simulink model "Lab1_adaptive"  (R2022b)
settings: Solver=VariableStepAuto  StartTime=0.0  StopTime=t  MaxStep=0.01  RelTol=1e-3
undefined symbols (not defined in the file): gamma, lambda, theta
settings Model: Creator=DuPont  LastModifiedBy=DuPont

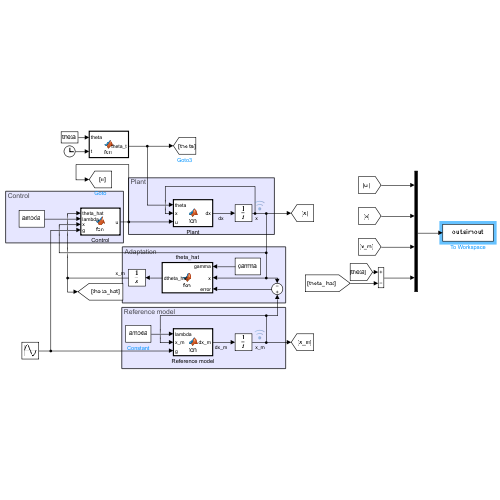
[thumbnail: Simulink's stored preview of the top-level diagram]
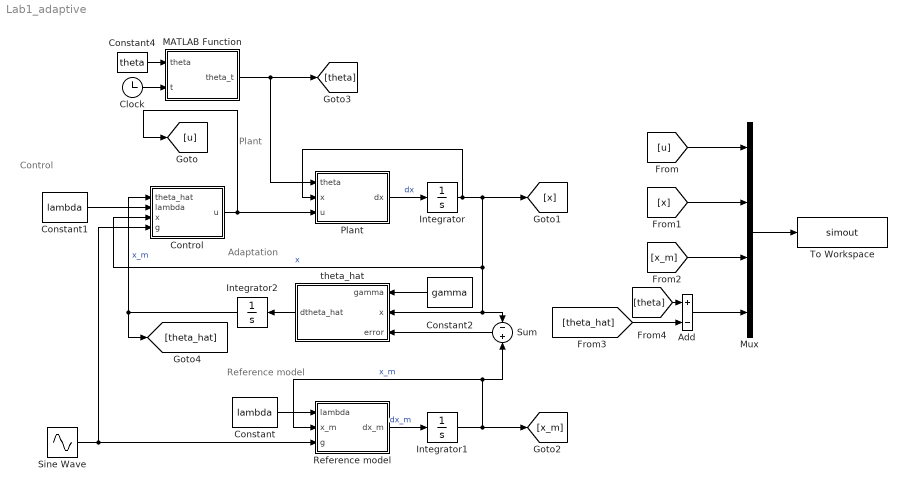
== system Lab1_adaptive ==
  note: Reference model
  note: Adaptation
  note: Control
  note: Plant
  Add : Sum  Inputs=+-
  Clock : Clock
  Constant : Constant  Value=lambda
  Constant1 : Constant  Value=lambda
  Constant2 : Constant  Value=gamma
  Constant4 : Constant  Value=theta
  Control : MATLAB Function  TreatAsAtomicUnit=on
  Integrator : Integrator
  Integrator1 : Integrator
  Integrator2 : Integrator
  MATLAB Function : MATLAB Function  TreatAsAtomicUnit=on
  Mux : Mux
  Plant : MATLAB Function  TreatAsAtomicUnit=on
  Reference model : MATLAB Function  TreatAsAtomicUnit=on
  Sine Wave : Sin  Bias=2  Frequency=8  SampleTime=0
  Sum : Sum  Inputs=-|+
  To Workspace : ToWorkspace  VariableName=simout  SaveFormat=Structure With Time  SampleTime=-1
  theta_hat : MATLAB Function  TreatAsAtomicUnit=on
  wires:
  Sine Wave/1 -> Reference model/3(g), Control/4(g)
  Control/1(u) -> [u], Plant/3(u)
  Plant/1(dx) -> Integrator/1  "dx"
  Integrator/1 -> Plant/2(x), [x], Control/3(x), theta_hat/2(x), Sum/1  "x"
  Reference model/1(dx_m) -> Integrator1/1  "dx_m"
  Integrator1/1 -> [x_m], Sum/2, Reference model/2(x_m)  "x_m"
  Constant/1 -> Reference model/1(lambda)
  Constant1/1 -> Control/2(lambda)
  Sum/1 -> theta_hat/3(error)
  Constant2/1 -> theta_hat/1(gamma)
  theta_hat/1(dtheta_hat) -> Integrator2/1
  Integrator2/1 -> [theta_hat], Control/1(theta_hat)  "x_m"
  MATLAB Function/1(theta_t) -> [theta], Plant/1(theta)
  [u] -> Mux/1
  [x] -> Mux/2
  [x_m] -> Mux/3
  Constant4/1 -> MATLAB Function/1(theta)
  Clock/1 -> MATLAB Function/2(t)
  [theta_hat] -> Add/2
  [theta] -> Add/1
  Add/1 -> Mux/4
  Mux/1 -> To Workspace/1

== matlab function Lab1_adaptive/Plant ==
  data: dx output; theta input; x input; u input
function dx = fcn(theta, x , u)

dx = theta*x + u;

== matlab function Lab1_adaptive/Control ==
  data: u output; theta_hat input; lambda input; x input; g input
function u = fcn(theta_hat, lambda, x, g)

u = -theta_hat*x - lambda*x + lambda*g;

== matlab function Lab1_adaptive/Reference model ==
  data: dx_m output; lambda input; x_m input; g input
function dx_m = fcn(lambda, x_m, g)

dx_m = -lambda*x_m + lambda*g;

== matlab function Lab1_adaptive/theta_hat ==
  data: dtheta_hat output; gamma input; x input; error input
function dtheta_hat  = fcn(gamma, x, error)

dtheta_hat = -gamma * x * error;

== matlab function Lab1_adaptive/MATLAB Function ==
  data: theta input; theta_t output; t input
function theta_t = fcn(theta, t)

if t < 10
    theta_t = theta;
else 
    theta_t = theta*3;
end
